simulink model "untitled"  (R2020b)
settings: Solver=FixedStepAuto  StartTime=0.0  StopTime=10.0  FixedStep=0.01  RelTol=1e-3
libraries: shared6dof x1, aerolibanim x1, aerolibadyn x1, aerolibatmos2 x1, aerolibasang x1
settings Model: Creator=jonas  LastModifiedBy=jonas

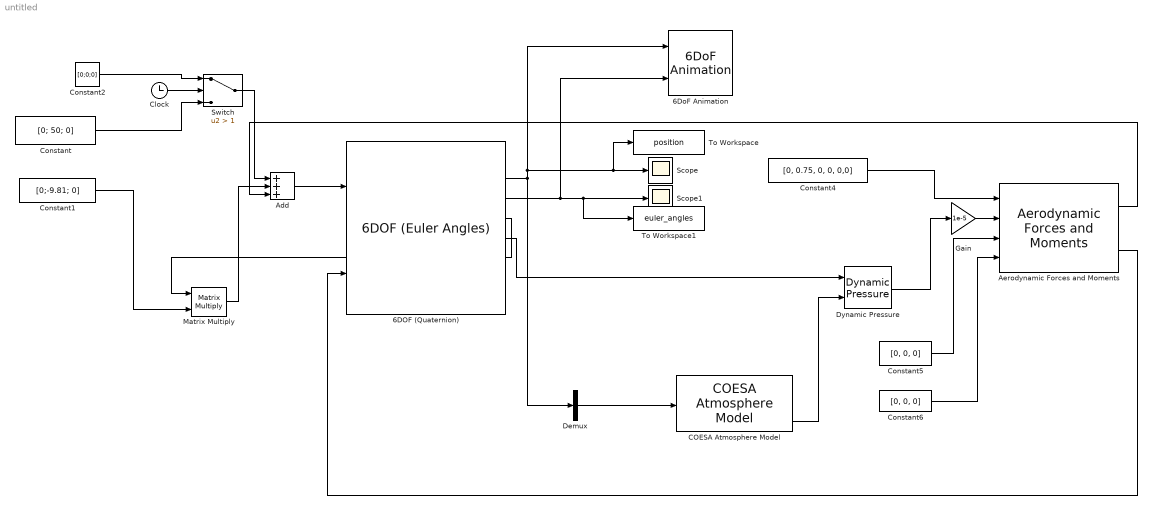
== system untitled ==
  6DOF (Quaternion) : shared6dof/6DOF (Euler Angles)  units=Metric (MKS)  mtype=Fixed  rep=Quaternion  xme_0=[0 0 0]  Vm_0=[0 0 0]  eul_0=[0 0 0.1]  pm_0=[0 0 0]  mass_0=2  mass_e=0.5  mass_f=2.0  inertia=I  inertia_e=eye(3)  inertia_f=2*eye(3)  k_quat=1.0  vre_flag=on  abi_flag=off  aMode=0  xme_statename=''  Vm_statename=''  eul_statename=''  quat_statename=''  pm_statename=''  mass_statename=''
      settings: SourceProductBaseCode=AE,PW,MT,UV,VE,VP
  6DoF Animation : aerolibanim/6DoF Animation  u1=[0 4000 -2000 2000 -5000 -3000]  u2=0.1  u3=1.0  u4=[4000 0 -5000]  u5=Fixed position  u6=[2000 500 -3150]  u7=10  u8=on
  Add : Sum  Inputs=+++
  "Aerodynamic Forces and Moments " : aerolibadyn/Aerodynamic Forces and Moments   inputAxes=Body  outputForceAxes=Body  outputMomentAxes=Body  S=0.314  b=0.1  cbar=1.5
  COESA Atmosphere Model : aerolibatmos2/COESA Atmosphere Model  units=Metric (MKS)  spec=1976 COESA-extended U.S. Standard Atmosphere  model=Profile  profile_var=High temperature  profile_percent=1%  profile_alt=5 km (16404 ft)  envelope_var=High temperature  envelope_percent=1%  action=Warning
  Clock : Clock
  Constant : Constant  Value=[0; 50; 0]
  Constant1 : Constant  Value=[0;-9.81; 0]
  Constant2 : Constant  Value=[0;0;0]
  Constant4 : Constant  Value=[0, 0.75, 0, 0, 0,0]
  Constant5 : Constant  Value=[0, 0, 0]
  Constant6 : Constant  Value=[0, 0, 0]
  Demux : Demux  Outputs=3
  Dynamic Pressure : aerolibasang/Dynamic Pressure
  Gain : Gain  Gain=1e-5
  Matrix Multiply : Product  Multiplication=Matrix(*)
  Scope : Scope
  Scope1 : Scope
  Switch : Switch  Criteria=u2 > Threshold  Threshold=1
  To Workspace : ToWorkspace  VariableName=position  SaveFormat=Timeseries  SampleTime=-1
  To Workspace1 : ToWorkspace  VariableName=euler_angles  SaveFormat=Timeseries  SampleTime=-1
  wires:
  Constant/1 -> Switch/3
  6DOF (Quaternion)/2 -> Demux/1, 6DoF Animation/1, To Workspace/1, Scope/1
  Constant1/1 -> Matrix Multiply/2
  Add/1 -> 6DOF (Quaternion)/1
  Clock/1 -> Switch/2
  Constant2/1 -> Switch/1
  Switch/1 -> Add/1
  6DOF (Quaternion)/5 -> Dynamic Pressure/1
  COESA Atmosphere Model/4 -> Dynamic Pressure/2
  Constant4/1 -> "Aerodynamic Forces and Moments "/1
  Constant5/1 -> "Aerodynamic Forces and Moments "/3
  Constant6/1 -> "Aerodynamic Forces and Moments "/4
  Demux/2 -> COESA Atmosphere Model/1
  Dynamic Pressure/1 -> Gain/1
  "Aerodynamic Forces and Moments "/2 -> 6DOF (Quaternion)/2
  "Aerodynamic Forces and Moments "/1 -> Add/3
  Gain/1 -> "Aerodynamic Forces and Moments "/2
  6DOF (Quaternion)/3 -> 6DoF Animation/2, To Workspace1/1, Scope1/1
  6DOF (Quaternion)/4 -> Matrix Multiply/1
  Matrix Multiply/1 -> Add/2
